simulink model "eq3_power_budget"  (R2025b)
settings: Solver=VariableStepAuto  StartTime=0.0  StopTime=10.0  RelTol=1e-3
undefined symbols (not defined in the file): T_INFER, T_SENSE, T_SLEEP, T_TX
settings Model: Creator=User  LastModifiedBy=User

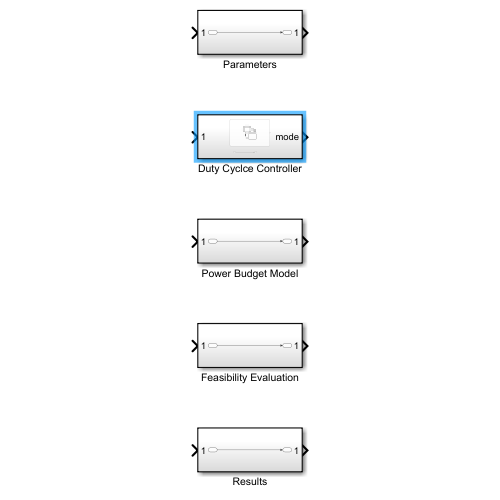
[thumbnail: Simulink's stored preview of the top-level diagram]
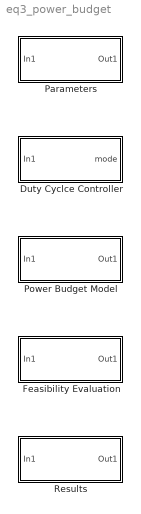
== system eq3_power_budget ==
  Duty Cyclce Controller : Subsystem
  Feasibility Evaluation : Subsystem
  Parameters : Subsystem
  Power Budget Model : Subsystem
  Results : Subsystem

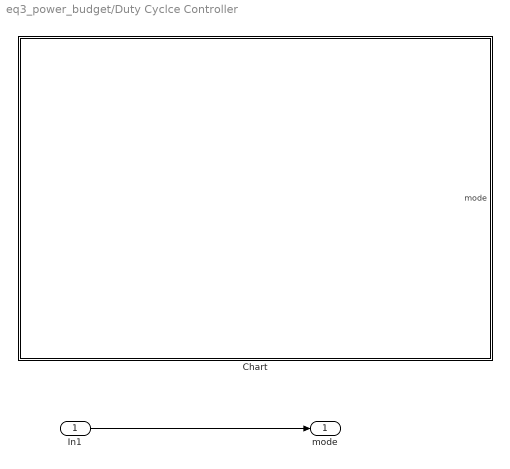
== system eq3_power_budget/Duty Cyclce Controller ==
  In1 : Inport
  Chart : Stateflow chart  TreatAsAtomicUnit=on
  mode : Outport
  wires:
  In1/1 -> mode/1

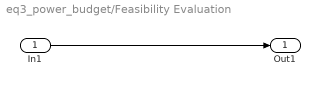
== system eq3_power_budget/Feasibility Evaluation ==
  In1 : Inport
  Out1 : Outport
  wires:
  In1/1 -> Out1/1

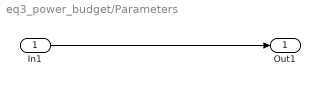
== system eq3_power_budget/Parameters ==
  In1 : Inport
  Out1 : Outport
  wires:
  In1/1 -> Out1/1

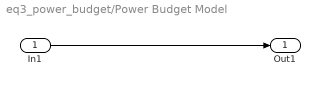
== system eq3_power_budget/Power Budget Model ==
  In1 : Inport
  Out1 : Outport
  wires:
  In1/1 -> Out1/1

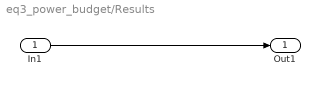
== system eq3_power_budget/Results ==
  In1 : Inport
  Out1 : Outport
  wires:
  In1/1 -> Out1/1

== stateflow chart eq3_power_budget/Duty Cyclce Controller/Chart ==
  state Sense
    entry:
    mode = 1;
  state Infer
    entry:
    mode = 2;
  state Sleep
    entry:
    mode = 4;
  state Transmit
    entry:
    mode = 3;
  (default) -> Sense
  Sense -> Infer : [after(T_SENSE,sec)]
  Sleep -> Sense : [after(T_SLEEP,sec)]
  Infer -> Transmit : [after(T_INFER,sec)]
  Transmit -> Sleep : [after(T_TX,sec)]
  data: T_SENSE parameter; T_SLEEP parameter; T_TX parameter; T_INFER parameter; mode output
